simulink model "case_14_mode_2_noise"  (R2025b)
settings: Solver=VariableStepAuto  StartTime=0.0  StopTime=10.0  RelTol=1e-3
settings Model: Creator=sanborkl  LastModifiedBy=sanborkl

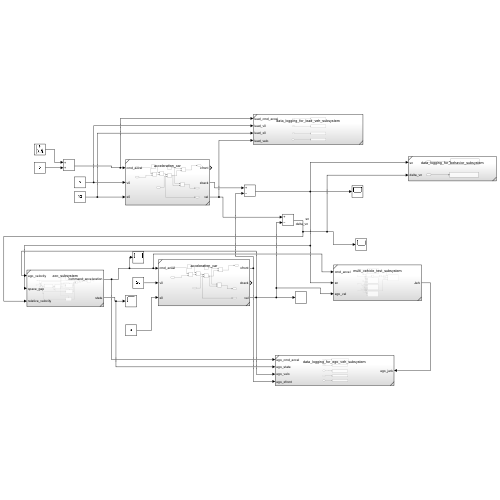
[thumbnail: Simulink's stored preview of the top-level diagram]
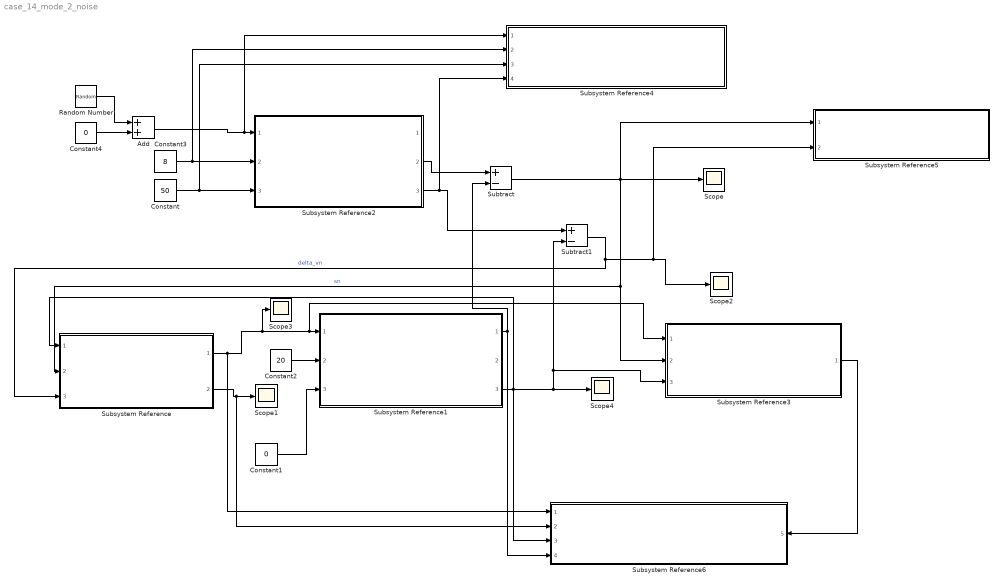
== system case_14_mode_2_noise ==
  Add : Sum
  Constant : Constant  Value=50
  Constant1 : Constant  Value=0
  Constant2 : Constant  Value=20
  Constant3 : Constant  Value=8
  Constant4 : Constant  Value=0
  Random Number : RandomNumber  Variance=0.005  SampleTime=0.1
  Scope{,1..4} (5 alike) : Scope
      Scope settings: ActiveDisplayYMinimum=-1  ActiveDisplayYMaximum=1
      Scope1 settings: ActiveDisplayYMinimum=-0.37499999999999989  ActiveDisplayYMaximum=3.375  DataLoggingVariableName=ScopeData2
      Scope2 settings: ActiveDisplayYMinimum=-10.624999999999998  ActiveDisplayYMaximum=95.625  DataLoggingVariableName=ScopeData3
      Scope3 settings: ActiveDisplayYMinimum=-0.4809516982343458  ActiveDisplayYMaximum=1.9609302395128785  DataLoggingVariableName=ScopeData4
      Scope4 settings: ActiveDisplayYMinimum=18.125  ActiveDisplayYMaximum=36.875
  Subsystem Reference : Subsystem  ReferencedSubsystem=acc_subsystem
  Subsystem Reference1 : Subsystem  ReferencedSubsystem=acceleration_car
  Subsystem Reference2 : Subsystem  ReferencedSubsystem=acceleration_car
  Subsystem Reference3 : Subsystem  ReferencedSubsystem=multi_vehicle_test_subsystem
  Subsystem Reference4 : Subsystem  ReferencedSubsystem=data_logging_for_lead_veh_subsystem
  Subsystem Reference5 : Subsystem  ReferencedSubsystem=data_logging_for_behavior_subsystem
  Subsystem Reference6 : Subsystem  ReferencedSubsystem=data_logging_for_ego_veh_subsystem
      settings: PortSchema="{\"entries\":[{\"content\":{\"sides\":[{\"content\":{\"connectorIds\":[\"In1\",\"In2\",\"In3\",\"In4\"]},\"type\":\"ConnectorPlacement.EquallySpacedRectSide\",\"uuid\":\"1bb3a8cf-f981-4f8a-aff9-03896ccf7d7c\"},{\"content\":{\"connectorIds\":[\"In5\"],\"side\":\"RIGHT\"},\"type\":\"ConnectorPlacement.EquallySpacedRectSide\",\"uuid\":\"3f6ac5cb-96be-44a3-8993-3635a91bd658\"},{\"content\":{\"side\":\"TOP\"},\"type\":\"ConnectorPlacement.EquallySpacedRectSide\",\"uuid\":\"c641fc7f-a424-4033-b273-2526f6b205c0\"}]},\"type\":\"ConnectorPlacement.EquallySpacedConnector\",\"uuid\":\"2a4be48e-084e-4aa6-b74f-8fe234fedc1a\"}],\"packageUris\":[\"http://schema.mathworks.com/mf0/Connector/R2020b\"],\"version\":\"1.0\"}"
  Subtract : Sum  Inputs=+-
  Subtract1 : Sum  Inputs=+-
  wires:
  Subsystem Reference2/2 -> Subtract/1
  Subtract1/1 -> Subsystem Reference5/2, Scope2/1, Subsystem Reference/3  "delta_vn"
  Subsystem Reference3/1 -> Subsystem Reference6/5
  Constant3/1 -> Subsystem Reference4/2, Subsystem Reference2/2
  Add/1 -> Subsystem Reference4/1, Subsystem Reference2/1
  Subsystem Reference/2 -> Subsystem Reference6/2, Scope1/1
  Random Number/1 -> Add/1
  Constant/1 -> Subsystem Reference4/3, Subsystem Reference2/3
  Constant4/1 -> Add/2
  Subsystem Reference/1 -> Subsystem Reference6/1, Scope3/1, Subsystem Reference3/1, Subsystem Reference1/1
  Constant2/1 -> Subsystem Reference1/2
  Constant1/1 -> Subsystem Reference1/3
  Subtract/1 -> Subsystem Reference5/1, Subsystem Reference3/2, Subsystem Reference/2, Scope/1  "sn"
  Subsystem Reference1/3 -> Subtract1/2, Subsystem Reference3/3, Scope4/1, Subsystem Reference6/3, Subsystem Reference/1
  Subsystem Reference2/3 -> Subsystem Reference4/4, Subtract1/1
  Subsystem Reference1/1 -> Subtract/2, Subsystem Reference6/4
